simulink model "lab10"  (R2017b)
settings: Solver=ode4  StartTime=0.0  StopTime=100  FixedStep=0.0001  RelTol=1e-3
settings Model: Creator=ayushi  LastModifiedBy=ayushi

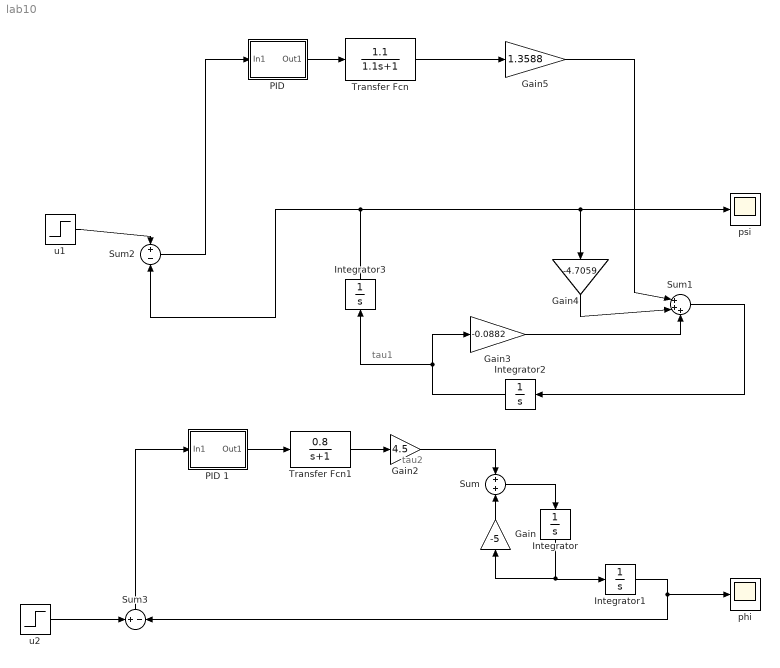
== system lab10 ==
  note: tau2
  note: tau1
  Gain : Gain  Gain=-5
  Gain2 : Gain  Gain=4.5
  Gain3 : Gain  Gain=-0.0882
  Gain4 : Gain  Gain=-4.7059
  Gain5 : Gain  Gain=1.3588
  Integrator{,1..3} (4 alike) : Integrator
  "PID " : Subsystem
  PID 1 : Subsystem
  Sum : Sum
  Sum1 : Sum  Inputs=|+++
  Sum2 : Sum  Inputs=+-
  Sum3 : Sum  Inputs=+-
  Transfer Fcn : TransferFcn  Numerator=[1.1]  Denominator=[1.1 1]
  Transfer Fcn1 : TransferFcn  Numerator=[0.8]  Denominator=[1 1]
  phi : Scope
  psi : Scope
  "u1 " : Step  After=1.57  SampleTime=0
  u2 : Step  SampleTime=0
  wires:
  Integrator3/1 -> psi/1, Gain4/1, Sum2/2
  Transfer Fcn/1 -> Gain5/1
  Gain/1 -> Sum/2
  Sum1/1 -> Integrator2/1
  Integrator2/1 -> Integrator3/1, Gain3/1
  Transfer Fcn1/1 -> Gain2/1
  Integrator/1 -> Integrator1/1, Gain/1
  Integrator1/1 -> Sum3/2, phi/1
  "PID "/1(Out1) -> Transfer Fcn/1
  Sum/1 -> Integrator/1
  PID 1/1(Out1) -> Transfer Fcn1/1
  Sum3/1 -> PID 1/1(In1)
  Gain2/1 -> Sum/1
  u2/1 -> Sum3/1
  "u1 "/1 -> Sum2/1
  Sum2/1 -> "PID "/1(In1)
  Gain3/1 -> Sum1/3
  Gain4/1 -> Sum1/2
  Gain5/1 -> Sum1/1

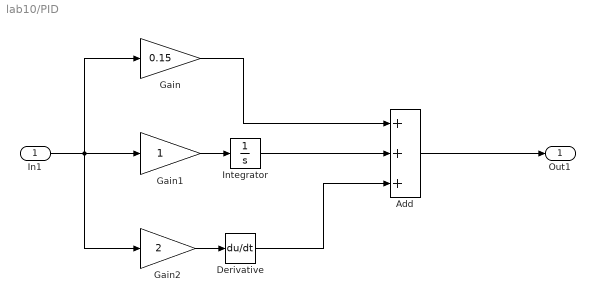
== system lab10/PID  ==
  In1 : Inport
  Add : Sum  Inputs=+++
  Derivative : Derivative
  Gain : Gain  Gain=0.15
  Gain1 : Gain
  Gain2 : Gain  Gain=2
  Integrator : Integrator
  Out1 : Outport
  wires:
  Gain/1 -> Add/1
  Gain2/1 -> Derivative/1
  Derivative/1 -> Add/3
  Integrator/1 -> Add/2
  Add/1 -> Out1/1
  In1/1 -> Gain2/1, Gain1/1, Gain/1
  Gain1/1 -> Integrator/1

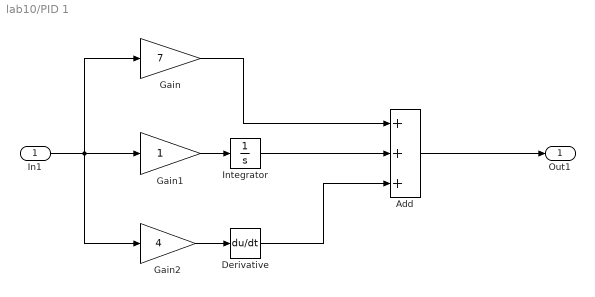
== system lab10/PID 1 ==
  In1 : Inport
  Add : Sum  Inputs=+++
  Derivative : Derivative
  Gain : Gain  Gain=7
  Gain1 : Gain
  Gain2 : Gain  Gain=4
  Integrator : Integrator
  Out1 : Outport
  wires:
  Gain/1 -> Add/1
  Gain2/1 -> Derivative/1
  Derivative/1 -> Add/3
  Integrator/1 -> Add/2
  Add/1 -> Out1/1
  In1/1 -> Gain2/1, Gain1/1, Gain/1
  Gain1/1 -> Integrator/1
